simulink model "sampleModel314"  (R2021b)
settings: Solver=VariableStepAuto  StartTime=0.0  StopTime=10.0  RelTol=1e-3
undefined symbols (not defined in the file or in its folder): DiscIntNeverNeededParam, Newton, Raphson
libraries: simulink x9, slpidlib x1
settings Model: Creator=user  LastModifiedBy=user

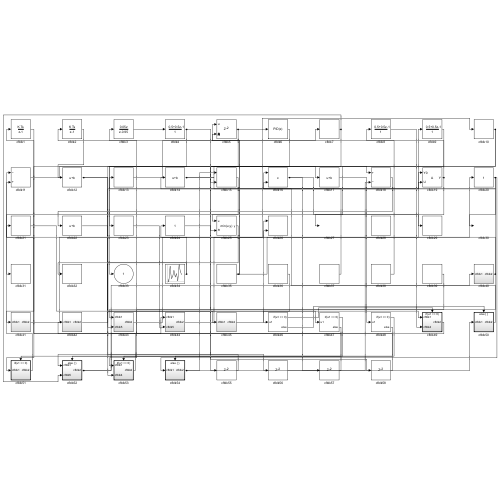
[thumbnail: Simulink's stored preview of the top-level diagram]
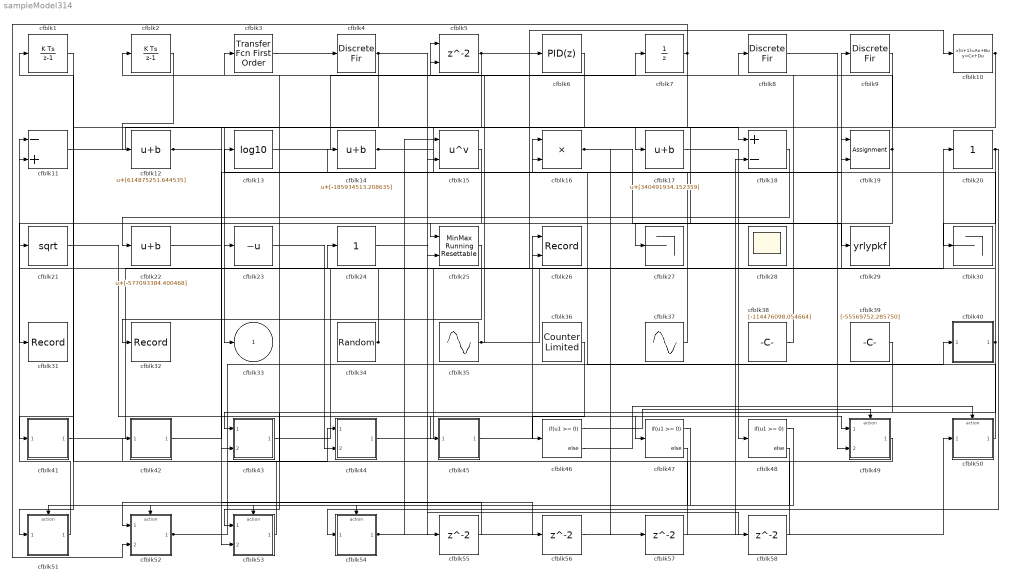
== system sampleModel314 ==
  cfblk1 : DiscreteIntegrator  ICPrevOutput=DiscIntNeverNeededParam  ICPrevScaledInput=DiscIntNeverNeededParam
  cfblk10 : DiscreteStateSpace
  cfblk11 : Sum  Inputs=-+
  cfblk12 : Bias  Bias=[614875251.644535]
  cfblk13 : Math  Operator=log10  SaturateOnIntegerOverflow=on
  cfblk14 : Bias  Bias=[-185934513.208635]
  cfblk15 : Math  Operator=pow  SaturateOnIntegerOverflow=on
  cfblk16 : Product
  cfblk17 : Bias  Bias=[340491934.152359]
  cfblk18 : Sum  Inputs=+-
  cfblk19 : Assignment  DiagnosticForDimensions=Warning  IndexOptions=Index vector (dialog)  Indices=1  OutputSizes=1
  cfblk2 : DiscreteIntegrator  ICPrevOutput=DiscIntNeverNeededParam  ICPrevScaledInput=DiscIntNeverNeededParam
  cfblk20 : simulink/Math Operations/Slider Gain  gain=1  low=0  high=2
  cfblk21 : Sqrt  SaturateOnIntegerOverflow=on
  cfblk22 : Bias  Bias=[-577093384.400468]
  cfblk23 : UnaryMinus
  cfblk24 : simulink/Math Operations/Slider Gain  gain=1  low=0  high=2
  cfblk25 : simulink/Math Operations/MinMax Running Resettable  Function=min  vinit=0.0
  cfblk26 : Record  FileSettingsInternal="{\"entries\":[{\"content\":{\"excelSettings\":{\"content\":{},\"type\":\"Streamout.ExcelSettings\"}},\"type\":\"Streamout.FileSettingStorage\",\"uuid\":\"386ec910-b54f-4735-98ac-f43c638e3766\"}],\"packageUris\":[\"http://schema.mathworks.com/mf0/streamout_blocks/R2020a\"],\"version\":\"1.0\"}"  Layout=[1 1]  SignalsInternal="{\"entries\":[{\"content\":{\"signals\":[{\"content\":{\"blockPath\":[\"sampleModel314/cfblk26\"],\"channel\":[],\"dimensions\":[1],\"domain\":\"sampleModel314/cfblk26\",\"lineColor\":\"#a2142f\",\"plots\":[1],\"port\":1,\"sid\":[\"\"],\"signalID\":13284,\"signalName\":\"cfblk45\"},\"type\":\"RecordBlkView.Signal\",\"uuid\":\"91ea6879-d668-42c6-b150-99f6e01f59d1\"},{\"content\":{\"blockPath\":[\"sampleModel314/cfblk26\"],\"channel\":[],\"dimensions\":[1],\"domain\":\"sampleModel314/cfblk26\",\"lineColor\":\"#139fff\",\"plots\":[1],\"port\":2,\"sid\":[\"\"],\"signalID\":13288,\"signalName\":\"cfblk43\"},\"type\":\"RecordBlkView.Signal\",\"uuid\":\"48596add-19b0-4b6d-b14f-700622423d45\"}]},\"type\":\"RecordBlkView.InputSignals\",\"uuid\":\"8c9e6b85-eeea-4281-886c-0a0be45bf9ce\"}],\"packageUris\":[\"http://schema.mathworks.com/mf0/streamout_blocks/R2020a\"],\"version\":\"1.0\"}"  VisualizationBindings="{\"xyplotplugin\":{\"info\":[{\"series\":[{\"bindingParametersList\":[{\"parameter\":\"X-Axis\",\"signalID\":13284,\"signalName\":\"cfblk45\"},{\"parameter\":\"Y-Axis\",\"signalID\":13288,\"signalName\":\"cfblk43\"}],\"seriesID\":27250}],\"subplotID\":1}]}}"  CompatibilityTag=XY
  cfblk27 : Terminator
  cfblk28 : Scope
      settings: Floating=on
  cfblk29 : ToWorkspace  VariableName=yrlypkf  SaveFormat=Timeseries  SampleTime=-1
  cfblk3 : simulink/Discrete/Transfer Fcn First Order  PoleZ=0.95  ICPrevOutput=0.0  DoSatur=off
  cfblk30 : Terminator
  cfblk31 : Record  FileSettingsInternal="{\"entries\":[{\"content\":{\"excelSettings\":{\"content\":{},\"type\":\"Streamout.ExcelSettings\"}},\"type\":\"Streamout.FileSettingStorage\",\"uuid\":\"19c1ac2f-acf3-4a07-95e7-987aae05738f\"}],\"packageUris\":[\"http://schema.mathworks.com/mf0/streamout_blocks/R2020a\"],\"version\":\"1.0\"}"  SignalsInternal="{\"entries\":[{\"content\":{\"signals\":[{\"content\":{\"blockPath\":[\"sampleModel314/cfblk31\"],\"channel\":[],\"dimensions\":[1],\"domain\":\"sampleModel314/cfblk31\",\"lineColor\":\"#b746ff\",\"plots\":[1],\"port\":1,\"sid\":[\"\"],\"signalID\":13292,\"signalName\":\"cfblk15\"},\"type\":\"RecordBlkView.Signal\",\"uuid\":\"b880eeeb-779d-40d8-845a-0423c84e336a\"}]},\"type\":\"RecordBlkView.InputSignals\",\"uuid\":\"3f360e8e-f8fe-4c28-aee0-a791d3f6d091\"}],\"packageUris\":[\"http://schema.mathworks.com/mf0/streamout_blocks/R2020a\"],\"version\":\"1.0\"}"  VisualizationBindings="{\"sparklinesplugin\":{\"info\":[{\"bindingParametersList\":[],\"subplotID\":1}]}}"
  cfblk32 : Record  FileSettingsInternal="{\"entries\":[{\"content\":{\"excelSettings\":{\"content\":{},\"type\":\"Streamout.ExcelSettings\"}},\"type\":\"Streamout.FileSettingStorage\",\"uuid\":\"19869da0-6022-4778-8006-6774d517005a\"}],\"packageUris\":[\"http://schema.mathworks.com/mf0/streamout_blocks/R2020a\"],\"version\":\"1.0\"}"  SignalsInternal="{\"entries\":[{\"content\":{\"signals\":[{\"content\":{\"blockPath\":[\"sampleModel314/cfblk32\"],\"channel\":[],\"dimensions\":[1],\"domain\":\"sampleModel314/cfblk32\",\"lineColor\":\"#64d413\",\"plots\":[1],\"port\":1,\"sid\":[\"\"],\"signalID\":13296,\"signalName\":\"cfblk34\"},\"type\":\"RecordBlkView.Signal\",\"uuid\":\"c962c7ba-9cef-44d1-b52b-9895dfb929df\"}]},\"type\":\"RecordBlkView.InputSignals\",\"uuid\":\"38e072ba-1e3d-4a13-b3d9-75eae7cbe8e1\"}],\"packageUris\":[\"http://schema.mathworks.com/mf0/streamout_blocks/R2020a\"],\"version\":\"1.0\"}"  VisualizationBindings="{\"sparklinesplugin\":{\"info\":[{\"bindingParametersList\":[],\"subplotID\":1}]}}"
  cfblk34 : UniformRandomNumber  Minimum=[-2547174862.064156]  Maximum=[737753289.405980]  Seed=[26097788.000000]  SampleTime=0.1
  cfblk35 : Sin  Amplitude=[-308332596.884744]  Bias=[-892118208.601684]  SampleTime=0
  cfblk36 : simulink/Sources/Counter Limited  uplimit=[753.000000]  tsamp=-1
  cfblk37 : Sin  Amplitude=[610076614.831349]  Bias=[166330221.537670]  SampleTime=0
  cfblk38 : Constant  Value=[-114476098.054664]  SampleTime=1
  cfblk39 : Constant  Value=[-55569752.285750]  SampleTime=1
  cfblk4 : DiscreteFir  SampleTime=1
  cfblk40 : Subsystem
  cfblk41 : Subsystem
  cfblk42 : Subsystem
  cfblk43 : Subsystem
  cfblk44 : Subsystem
  cfblk45 : Subsystem
  cfblk46 : If  IfExpression=u1 >= 0  SampleTime=1
  cfblk47 : If  IfExpression=u1 >= 0  SampleTime=1
  cfblk48 : If  IfExpression=u1 >= 0  SampleTime=1
  cfblk49 : Subsystem  TreatAsAtomicUnit=on
  cfblk5 : Delay  ShowEnablePort=on  SampleTime=1
      settings: InputPortMap=u0,e6
  cfblk50 : Subsystem  TreatAsAtomicUnit=on
  cfblk51 : Subsystem  TreatAsAtomicUnit=on
  cfblk52 : Subsystem  TreatAsAtomicUnit=on
  cfblk53 : Subsystem  TreatAsAtomicUnit=on
  cfblk54 : Subsystem  TreatAsAtomicUnit=on
  cfblk{55..58} (4 alike) : Delay  SampleTime=1
  cfblk6 : slpidlib/PID Controller  Controller=PID  Form=Parallel  TimeDomain=Discrete-time  UseExternalTs=off  SampleTime=1  IntegratorMethod=Forward Euler  FilterMethod=Forward Euler  ControllerParametersSource=internal  P=1  I=1  D=0  UseFilter=on  N=100  TunerSelectOption=Transfer Function Based (PID Tuner App)  InitialConditionSource=internal  InitialConditionForIntegrator=0  InitialConditionForFilter=0  DifferentiatorICPrevScaledInput=0  ExternalReset=none  TrackingMode=off  Kt=1  LimitOutput=off  SatLimitsSource=internal  UpperSaturationLimit=inf  LowerSaturationLimit=-inf  LinearizeAsGain=off  AntiWindupMode=none  Kb=1  POutMin=[]  POutMax=[]  IOutMin=[]  IOutMax=[]  DOutMin=[]  DOutMax=[]  NOutMin=[]  NOutMax=[]  SumOutMin=[]  SumOutMax=[]  SaturationOutMin=[]  SaturationOutMax=[]  PParamMin=[]  PParamMax=[]  IParamMin=[]  IParamMax=[]  DParamMin=[]  DParamMax=[]  NParamMin=[]  NParamMax=[]  KbParamMin=[]  KbParamMax=[]  KtParamMin=[]  KtParamMax=[]  KbOutMin=[]  KbOutMax=[]  KtOutMin=[]  KtOutMax=[]  IntegratorOutMin=[]  IntegratorOutMax=[]  FilterOutMin=[]  FilterOutMax=[]  SumI1OutMin=[]  SumI1OutMax=[]  SumI2OutMin=[]  SumI2OutMax=[]  SumI3OutMin=[]  SumI3OutMax=[]  SumI4OutMin=[]  SumI4OutMax=[]  SumDOutMin=[]  SumDOutMax=[]  DifferentiatorOutMin=[]  DifferentiatorOutMax=[]  FilterDiffOutCoefMin=[]  FilterDiffOutCoefMax=[]  ReciprocalOutMin=[]  ReciprocalOutMax=[]  SumDenOutMin=[]  SumDenOutMax=[]  SumNumOutMin=[]  SumNumOutMax=[]  DivideOutMin=[]  DivideOutMax=[]  UdiffTsProdOutMin=[]  UdiffTsProdOutMax=[]  NTsProdOutMin=[]  NTsProdOutMax=[]  UintegralTsProdOutMin=[]  UintegralTsProdOutMax=[]  UngainTsProdOutMin=[]  UngainTsProdOutMax=[]  IntegratorContinuousStateAttributes=''  IntegratorStateMustResolveToSignalObject=off  IntegratorRTWStateStorageClass=Auto  FilterContinuousStateAttributes=''  FilterStateMustResolveToSignalObject=off  FilterRTWStateStorageClass=Auto  ParallelPVariant=InternalParameters  IdealPVariant=Disabled  IVariant=InternalParameters  DVariant=InternalParameters  IntegratorVariant=Discrete  SatVariant=Disabled  AWVariant=Passthrough  PCopyVariant=Disabled  TRVariant=Disabled  FdbkBlocksVariant=Forward  IdealPFdbkVariant=Disabled  SatFdbkVariant=Disabled  DerivativeFilterVariant=ForwardEulerFilter  NVariant=InternalParameters  NCopyVariant=Disabled  FilterICVariant=InternalICsFilter  IntegratorICVariant=InternalICs  ExternalResetVariant=Disabled  TRSumVariant=Passthrough  SumFdbkVariant=Disabled  SumVariant=Sum_PID  TsampFilterVariant=InternalTs  TsampNgainVariant=Passthrough  TsampIntegralVariant=Passthrough  ExternalSaturationOutDataTypeStr=Inherit: Same as second input
  cfblk7 : UnitDelay  HasFrameUpgradeWarning=on
  cfblk8 : DiscreteFir  SampleTime=1
  cfblk9 : DiscreteFir  SampleTime=1
  cfblk33 : Outport
  wires:
  cfblk52/1(cfblk2) -> cfblk40/1(cfblk1), cfblk44/1(cfblk1)
  cfblk19/1 -> cfblk25/1, cfblk2/1
  cfblk34/1 -> cfblk11/1, cfblk32/1
  cfblk3/1 -> cfblk4/1
  cfblk51/1(cfblk2) -> cfblk11/2
  cfblk20/1 -> cfblk54/1(cfblk1), cfblk30/1, cfblk16/2
  cfblk44/1(cfblk2) -> cfblk9/1
  cfblk18/1 -> cfblk22/1
  cfblk9/1 -> cfblk33/1
  cfblk11/1 -> cfblk18/1
  cfblk6/1 -> cfblk23/1
  cfblk15/1 -> cfblk31/1
  cfblk45/1(cfblk2) -> cfblk26/1
  cfblk36/1 -> cfblk46/1
  cfblk39/1 -> cfblk43/1(cfblk1)
  cfblk37/1 -> cfblk13/1
  cfblk38/1 -> cfblk8/1
  cfblk12/1 -> cfblk44/2(cfblk5), cfblk56/1
  cfblk22/1 -> cfblk45/1(cfblk1)
  cfblk5/1 -> cfblk25/2, cfblk10/1
  cfblk1/1 -> cfblk41/1(cfblk1)
  cfblk43/1(cfblk2) -> cfblk26/2
  cfblk40/1(cfblk2) -> cfblk24/1, cfblk14/1, cfblk53/1(cfblk1)
  cfblk2/1 -> cfblk12/1
  cfblk21/1 -> cfblk49/1(cfblk1)
  cfblk35/1 -> cfblk20/1, cfblk5/1, cfblk5/2
  cfblk17/1 -> cfblk48/1
  cfblk53/1(cfblk2) -> cfblk21/1
  cfblk14/1 -> cfblk17/1, cfblk19/2
  cfblk4/1 -> cfblk53/2(cfblk4), cfblk58/1
  cfblk13/1 -> cfblk7/1
  cfblk7/1 -> cfblk52/2(cfblk5), cfblk15/2
  cfblk10/1 -> cfblk51/1(cfblk1), cfblk27/1
  cfblk16/1 -> cfblk29/1, cfblk57/1
  cfblk23/1 -> cfblk47/1
  cfblk42/1(cfblk2) -> cfblk19/1
  cfblk54/1(cfblk2) -> cfblk18/2, cfblk15/1
  cfblk50/1(cfblk2) -> cfblk16/1
  cfblk25/1 -> cfblk43/2(cfblk5)
  cfblk41/1(cfblk2) -> cfblk6/1
  cfblk8/1 -> cfblk49/2(cfblk4)
  cfblk49/1(cfblk2) -> cfblk42/1(cfblk1)
  cfblk46/1 -> cfblk49/Action
  cfblk46/2 -> cfblk50/Action
  cfblk47/1 -> cfblk51/Action
  cfblk47/2 -> cfblk52/Action
  cfblk48/1 -> cfblk53/Action
  cfblk48/2 -> cfblk54/Action
  cfblk24/1 -> cfblk55/1
  cfblk55/1 -> cfblk52/1(cfblk1)
  cfblk56/1 -> cfblk50/1(cfblk1)
  cfblk57/1 -> cfblk1/1
  cfblk58/1 -> cfblk3/1

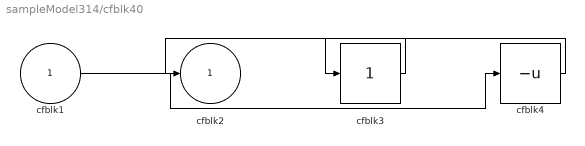
== system sampleModel314/cfblk40 ==
  cfblk1 : Inport
  cfblk3 : simulink/Math Operations/Slider Gain  gain=1  low=0  high=2
  cfblk4 : UnaryMinus
  cfblk2 : Outport
  wires:
  cfblk4/1 -> cfblk3/1
  cfblk1/1 -> cfblk4/1
  cfblk3/1 -> cfblk2/1

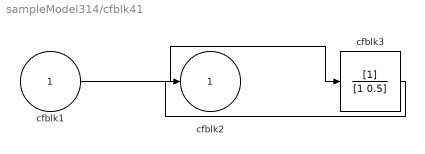
== system sampleModel314/cfblk41 ==
  cfblk1 : Inport
  cfblk3 : DiscreteFilter  SampleTime=1
  cfblk2 : Outport
  wires:
  cfblk1/1 -> cfblk3/1
  cfblk3/1 -> cfblk2/1

== system sampleModel314/cfblk42 ==
  cfblk1 : Inport
  cfblk3 : DotProduct  InputSameDT=on  OutDataTypeStr=Inherit: Inherit via internal rule
  cfblk2 : Outport
  wires:
  cfblk1/1 -> cfblk3/1, cfblk3/2
  cfblk3/1 -> cfblk2/1

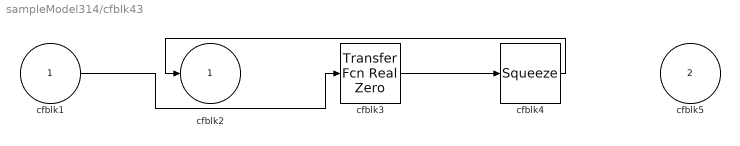
== system sampleModel314/cfblk43 ==
  cfblk1 : Inport
  cfblk5 : Inport  Port=2
  cfblk3 : simulink/Discrete/Transfer Fcn Real Zero  ZeroZ=0.75  ICPrevInput=0.0  DoSatur=off
      settings: SourceProductBaseCode=SL
  cfblk4 : Squeeze
  cfblk2 : Outport
  wires:
  cfblk4/1 -> cfblk2/1
  cfblk1/1 -> cfblk3/1
  cfblk3/1 -> cfblk4/1

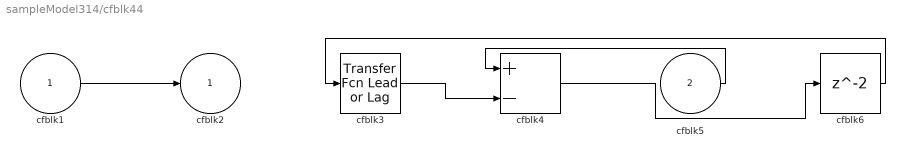
== system sampleModel314/cfblk44 ==
  cfblk1 : Inport
  cfblk5 : Inport  Port=2
  cfblk3 : simulink/Discrete/Transfer Fcn Lead or Lag  PoleZ=0.95  ZeroZ=0.75  ICPrevOutput=0.0  ICPrevInput=0.0  DoSatur=off
      settings: SourceProductBaseCode=SL
  cfblk4 : Sum  Inputs=+-
  cfblk6 : Delay  SampleTime=1
  cfblk2 : Outport
  wires:
  cfblk5/1 -> cfblk4/1
  cfblk3/1 -> cfblk4/2
  cfblk1/1 -> cfblk2/1
  cfblk4/1 -> cfblk6/1
  cfblk6/1 -> cfblk3/1

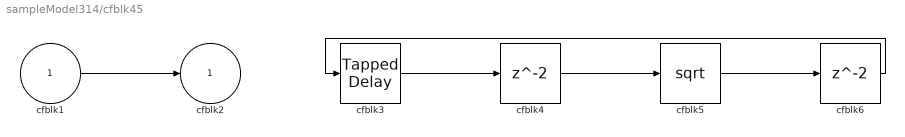
== system sampleModel314/cfblk45 ==
  cfblk1 : Inport
  cfblk3 : simulink/Discrete/Tapped Delay  vinit=0.0  samptime=-1  NumDelays=1  DelayOrder=Oldest  includeCurrent=off
  cfblk4 : Delay  SampleTime=1
  cfblk5 : Sqrt  SaturateOnIntegerOverflow=on
  cfblk6 : Delay  SampleTime=1
  cfblk2 : Outport
  wires:
  cfblk1/1 -> cfblk2/1
  cfblk4/1 -> cfblk5/1
  cfblk3/1 -> cfblk4/1
  cfblk5/1 -> cfblk6/1
  cfblk6/1 -> cfblk3/1

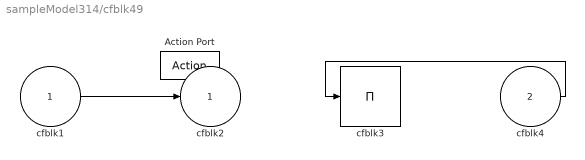
== system sampleModel314/cfblk49 ==
  cfblk1 : Inport
  cfblk4 : Inport  Port=2
  Action Port : ActionPort  ActionPortLabel=if(u1 >= 0)
  cfblk3 : Product  Inputs=*
  cfblk2 : Outport
  wires:
  cfblk1/1 -> cfblk2/1
  cfblk4/1 -> cfblk3/1

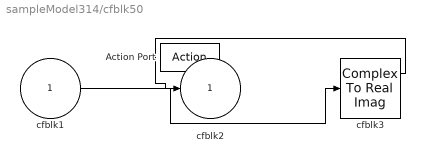
== system sampleModel314/cfblk50 ==
  cfblk1 : Inport
  Action Port : ActionPort  ActionPortLabel=else
  cfblk3 : ComplexToRealImag
  cfblk2 : Outport
  wires:
  cfblk1/1 -> cfblk3/1
  cfblk3/1 -> cfblk2/1

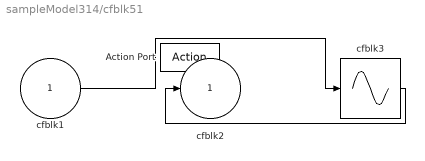
== system sampleModel314/cfblk51 ==
  cfblk1 : Inport
  Action Port : ActionPort  ActionPortLabel=if(u1 >= 0)
  cfblk3 : Sin  TimeSource=Use external signal  SampleTime=0
  cfblk2 : Outport
  wires:
  cfblk3/1 -> cfblk2/1
  cfblk1/1 -> cfblk3/1

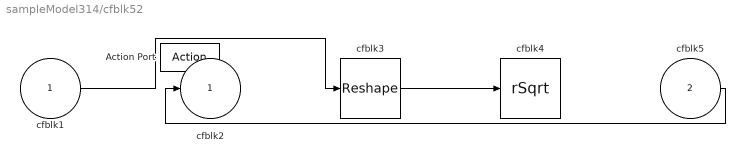
== system sampleModel314/cfblk52 ==
  cfblk1 : Inport
  cfblk5 : Inport  Port=2
  Action Port : ActionPort  ActionPortLabel=else
  cfblk3 : Reshape
  cfblk4 : Sqrt  Operator=rSqrt  AlgorithmType=Newton-Raphson  SaturateOnIntegerOverflow=on
  cfblk2 : Outport
  wires:
  cfblk5/1 -> cfblk2/1
  cfblk1/1 -> cfblk3/1
  cfblk3/1 -> cfblk4/1

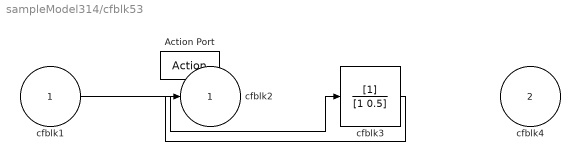
== system sampleModel314/cfblk53 ==
  cfblk1 : Inport
  cfblk4 : Inport  Port=2
  Action Port : ActionPort  ActionPortLabel=if(u1 >= 0)
  cfblk3 : DiscreteFilter
  cfblk2 : Outport
  wires:
  cfblk1/1 -> cfblk3/1
  cfblk3/1 -> cfblk2/1

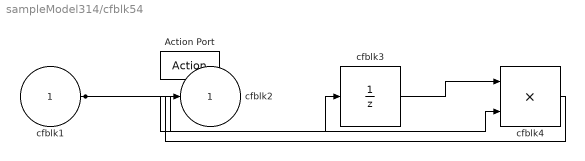
== system sampleModel314/cfblk54 ==
  cfblk1 : Inport
  Action Port : ActionPort  ActionPortLabel=else
  cfblk3 : UnitDelay  SampleTime=-1  HasFrameUpgradeWarning=on
  cfblk4 : Product  Inputs=**
  cfblk2 : Outport
  wires:
  cfblk3/1 -> cfblk4/1
  cfblk1/1 -> cfblk3/1, cfblk4/2
  cfblk4/1 -> cfblk2/1
